simulink model "dstatcom_avg"  (Simulink 7.9)
settings: Solver=ode23tb  SolverMode=SingleTasking  StartTime=0.0  StopTime=12  FixedStep=Ts  MaxStep=1/60  RelTol=1e-4
InitFcn:
  | Ts=40e-6;
  | tic;
StopFcn:
  | toc;
undefined symbols (not defined in the file or in its folder): D11, Delta, DiscIntNeverNeededParam
libraries: powerlib x53, powerlib_extras x39
(part 2 of 2)

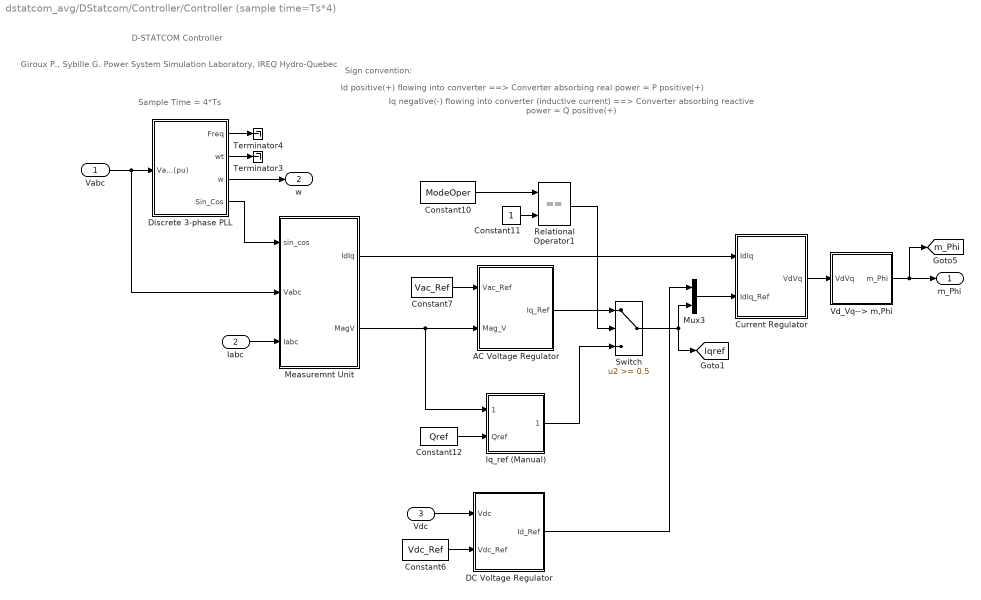
== system dstatcom_avg/DStatcom/Controller/Controller (sample time=Ts*4) ==
  note: D-STATCOM Controller
  note: Giroux P., Sybille G.
      | Power System Simulation Laboratory, IREQ
      | Hydro-Quebec
  note: Iq negative(-) flowing into converter (inductive current) ==> Converter absorbing reactive power = Q positive(+)
  note: Sign convention:
  note: Id positive(+) flowing into converter ==> Converter absorbing real power = P positive(+)
  note: Sample Time = 4*Ts
  Vabc : Inport  PortDimensions=3
  Iabc : Inport  Port=2  PortDimensions=3
  Vdc : Inport  Port=3  PortDimensions=1
  AC Voltage Regulator : Subsystem  mask(DC Voltage regulator){Kp=Kp_Vac, Ki=Ki_Vac, Ts=4*Ts}
      mask prompts: Kp "Proportional gain (Kp):"; Ki "Integral gain(Ki)"; Ts "Sample time:"
  Constant10 : Constant  Value=ModeOper
  Constant11 : Constant
  Constant12 : Constant  Value=Qref
  Constant6 : Constant  Value=Vdc_Ref
  Constant7 : Constant  Value=Vac_Ref
  Current Regulator : Subsystem  mask(Current Regulators){Kp=Kp_I, Ki=Ki_I, Kd=Kd_I, TcD=0.2e-3, Par_Limits=[1 -1], Init=0, Ts=4*Ts}
      mask prompts: Kp "Proportional gain (Kp):"; Ki "Integral gain (Ki):"; Kd "Derivative gain (Kd):"; TcD "Time constant for derivative (s):"; Par_Limits "Output limits: [ Upper   Lower ]"; Init "Output initial value:"; Ts "Sample time:"
      mask help:
      | Sign convention:
      | Id positive(+) flowing into converter ==> Converter absorbing real power = P positive(+)
      | Iq negative(-) flowing into converter (inductive current) ==> Converter absorbing reactive power = Q positive(+)
  DC Voltage Regulator : Subsystem  mask(DC Voltage regulator){Kp=Kp_Vdc, Ki=Ki_Vdc, Ts=4*Ts}
      mask prompts: Kp "Proportional gain (Kp):"; Ki "Integral gain(Ki)"; Ts "Sample time:"
  Discrete 3-phase PLL : Subsystem  mask(Discrete 3-phase PLL){Par_Init=[3.7 60], ParK=[60 1400], Ts=4*Ts}
      mask prompts: Par_Init "Initial inputs:[ Phase(degrees)   Frequency(Hz) ]"; ParK "Regulator gains [ Kp  Ki ]"; Ts "Sample time:"
      mask help:
      | This Phase Locked Loop (PLL) system can be used  to synchronize on a set of variable frequency, three-phase sinusoidal signals.
      |
      | Input 1: Vector containing the normalized
      |              three-phase signals [Va Vb Vc]
      | Output 1:  Measured frequency (Hz) = w/(2pi)
      | Output 2:  Ramp w.t   varying between  0 and 2*pi,
      | synchronized on zero crossings of the fundamental (positive-sequence) of phase A.
      | Output 3: Vector [sin(wt) cos(wt)]
      mask init:
      | Kp=ParK(1);
      | Ki=ParK(2);
      | Phase_Init=Par_Init(1);
      | Finit=Par_Init(2);
  Iq_ref (Manual) : Subsystem
  Measuremnt Unit : Subsystem
  Mux3 : Mux  Inputs=2
  Relational Operator1 : RelationalOperator  Operator===  InputSameDT=on
  Switch : Switch  Threshold=0.5  SaturateOnIntegerOverflow=on  InputSameDT=on
  Terminator3 : Terminator
  Terminator4 : Terminator
  Vd_Vq--> m,Phi : Subsystem
  m_Phi : Outport
  w : Outport  Port=2
  tag scope: Iqref=global, m_Phi=global
  wires:
  Vd_Vq--> m,Phi/1(m_Phi) -> [m_Phi], m_Phi/1
  Current Regulator/1(VdVq) -> Vd_Vq--> m,Phi/1(VdVq)
  Relational Operator1/1 -> Switch/2
  Iq_ref (Manual)/1(Iqref*) -> Switch/3
  DC Voltage Regulator/1(Id_Ref) -> Mux3/1
  Switch/1 -> [Iqref], Mux3/2
  Mux3/1 -> Current Regulator/2(IdIq_Ref)
  AC Voltage Regulator/1(Iq_Ref) -> Switch/1
  Measuremnt Unit/1(IdIq) -> Current Regulator/1(IdIq)
  Constant7/1 -> AC Voltage Regulator/1(Vac_Ref)
  Measuremnt Unit/2(MagV) -> Iq_ref (Manual)/1(MagV), AC Voltage Regulator/2(Mag_V)
  Iabc/1 -> Measuremnt Unit/3(Iabc)
  Discrete 3-phase PLL/4(Sin_Cos) -> Measuremnt Unit/1(sin_cos)
  Discrete 3-phase PLL/3(w) -> w/1
  Discrete 3-phase PLL/1(Freq) -> Terminator4/1
  Discrete 3-phase PLL/2(wt) -> Terminator3/1
  Constant12/1 -> Iq_ref (Manual)/2(Qref)
  Constant10/1 -> Relational Operator1/1
  Constant11/1 -> Relational Operator1/2
  Vdc/1 -> DC Voltage Regulator/1(Vdc)
  Constant6/1 -> DC Voltage Regulator/2(Vdc_Ref)
  Vabc/1 -> Measuremnt Unit/2(Vabc), Discrete 3-phase PLL/1(Vabc (pu))

== system dstatcom_avg/DStatcom/Controller/m_Phi->Vabc(t) ==
  m_Phi : Inport
  theta : Inport  Port=2
  Constant1 : Constant  Value=[0 -2*pi/3 2*pi/3]
  Demux : Demux  Outputs=2
  Product2 : Product  SaturateOnIntegerOverflow=on  InputSameDT=on  OutDataTypeStr=Inherit: Same as first input
  Sum4 : Sum  Inputs=+++  SaturateOnIntegerOverflow=on  InputSameDT=on  OutDataTypeStr=Inherit: Same as first input
  Trigonometric Function1 : Trigonometry
  deg. ->rad : Gain  Gain=pi/180  SaturateOnIntegerOverflow=on  OutDataTypeStr=Inherit: Same as input  ParamDataTypeStr=Inherit: Same as input
  Vabc (t) : Outport
  wires:
  Demux/2 -> deg. ->rad/1
  theta/1 -> Sum4/3
  deg. ->rad/1 -> Sum4/1
  m_Phi/1 -> Demux/1
  Product2/1 -> Vabc (t)/1
  Demux/1 -> Product2/1
  Constant1/1 -> Sum4/2
  Sum4/1 -> Trigonometric Function1/1
  Trigonometric Function1/1 -> Product2/2

== system dstatcom_avg/DStatcom/Controller/w->theta ==
  w : Inport
  Constant4 : Constant  Value=2*pi
  Discrete-Time Integrator : DiscreteIntegrator  SampleTime=Ts  ICPrevOutput=DiscIntNeverNeededParam  ICPrevScaledInput=DiscIntNeverNeededParam
  Math Function : Math  Operator=mod  SaturateOnIntegerOverflow=on
  theta : Outport
  wires:
  Math Function/1 -> theta/1
  w/1 -> Discrete-Time Integrator/1
  Constant4/1 -> Math Function/2
  Discrete-Time Integrator/1 -> Math Function/1

== system dstatcom_avg/DStatcom/Controller/Controller (sample time=Ts*4)/AC Voltage Regulator ==
  Vac_Ref : Inport
  Mag_V : Inport  Port=2
  Discrete PI Controller : powerlib_extras/Discrete  Control Blocks/Discrete PI Controller  Kp=Kp  Ki=Ki  Par_Limits=[1 -1]  Init=0  Ts=Ts
  Sum : Sum  Inputs=|+-  SaturateOnIntegerOverflow=on  InputSameDT=on  OutDataTypeStr=Inherit: Same as first input
  Iq_Ref : Outport  InitialOutput=0
  wires:
  Sum/1 -> Discrete PI Controller/1
  Vac_Ref/1 -> Sum/1
  Mag_V/1 -> Sum/2
  Discrete PI Controller/1 -> Iq_Ref/1

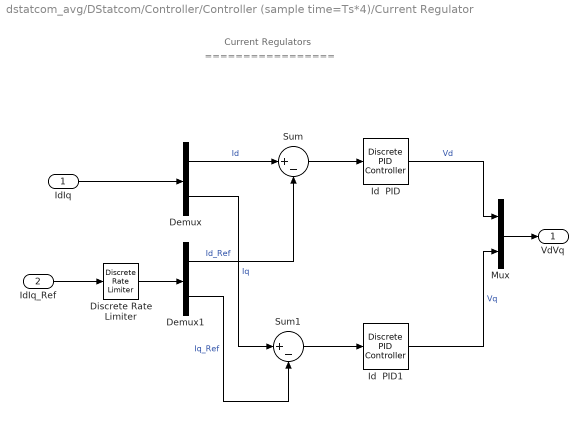
== system dstatcom_avg/DStatcom/Controller/Controller (sample time=Ts*4)/Current Regulator ==
  note: =================
  note: Current Regulators
  IdIq : Inport  PortDimensions=2
  IdIq_Ref : Inport  Port=2  PortDimensions=2
  Demux : Demux  Outputs=2
  Demux1 : Demux  Outputs=2
  Discrete Rate Limiter : powerlib_extras/Discrete  Control Blocks/Discrete Rate Limiter  R=240  F=-240  Vinit=0  Ts=Ts
  Id  PID : powerlib_extras/Discrete  Control Blocks/Discrete PID Controller  Kp=Kp  Ki=Ki  Kd=Kd  TcD=TcD  Par_Limits=Par_Limits  Init=Init  Ts=Ts
  Id  PID1 : powerlib_extras/Discrete  Control Blocks/Discrete PID Controller  Kp=Kp  Ki=Ki  Kd=Kd  TcD=TcD  Par_Limits=Par_Limits  Init=Init  Ts=Ts
  Mux : Mux  Inputs=2
  Sum : Sum  Inputs=|+-  SaturateOnIntegerOverflow=on  InputSameDT=on  OutDataTypeStr=Inherit: Same as first input
  Sum1 : Sum  Inputs=|+-  SaturateOnIntegerOverflow=on  InputSameDT=on  OutDataTypeStr=Inherit: Same as first input
  VdVq : Outport
  wires:
  Discrete Rate Limiter/1 -> Demux1/1
  IdIq_Ref/1 -> Discrete Rate Limiter/1
  Mux/1 -> VdVq/1
  Sum/1 -> Id  PID/1
  Demux1/2 -> Sum1/2  "Iq_Ref"
  Sum1/1 -> Id  PID1/1
  Demux/2 -> Sum1/1  "Iq"
  Demux1/1 -> Sum/2  "Id_Ref"
  Demux/1 -> Sum/1  "Id"
  Id  PID/1 -> Mux/1  "Vd"
  Id  PID1/1 -> Mux/2  "Vq"
  IdIq/1 -> Demux/1

== system dstatcom_avg/DStatcom/Controller/Controller (sample time=Ts*4)/DC Voltage Regulator ==
  Vdc : Inport
  Vdc_Ref : Inport  Port=2
  -1<Id<+1 : Saturate  UpperLimit=1  LowerLimit=-1
  2250<Vdc<3750 : Saturate  UpperLimit=3750  LowerLimit=2250
  Discrete PI Controller : powerlib_extras/Discrete  Control Blocks/Discrete PI Controller  Kp=Kp  Ki=Ki  Par_Limits=[1 -1]  Init=0  Ts=Ts
  Discrete Rate Limiter1 : powerlib_extras/Discrete  Control Blocks/Discrete Rate Limiter  R=10000  F=-10000  Vinit=3000  Ts=Ts
  Sum : Sum  Inputs=|+-  SaturateOnIntegerOverflow=on  InputSameDT=on  OutDataTypeStr=Inherit: Same as first input
  Id_Ref : Outport  InitialOutput=0
  wires:
  Vdc_Ref/1 -> 2250<Vdc<3750/1
  2250<Vdc<3750/1 -> Discrete Rate Limiter1/1
  Sum/1 -> Discrete PI Controller/1
  Vdc/1 -> Sum/2
  Discrete Rate Limiter1/1 -> Sum/1
  Discrete PI Controller/1 -> -1<Id<+1/1
  -1<Id<+1/1 -> Id_Ref/1

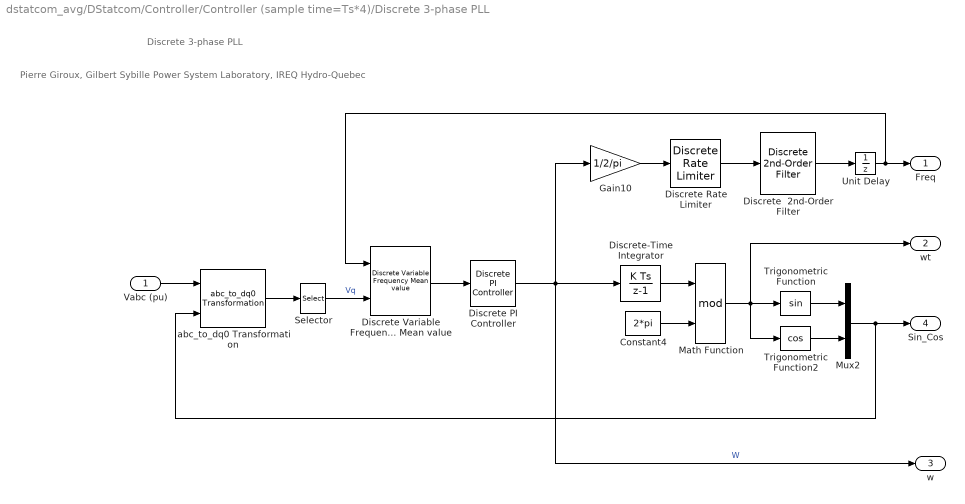
== system dstatcom_avg/DStatcom/Controller/Controller (sample time=Ts*4)/Discrete 3-phase PLL ==
  note: Discrete 3-phase PLL
  note: Pierre Giroux, Gilbert Sybille
      | Power System Laboratory, IREQ
      | Hydro-Quebec
  Vabc (pu) : Inport  PortDimensions=3
  Constant4 : Constant  Value=2*pi
  Discrete PI Controller : powerlib_extras/Discrete  Control Blocks/Discrete PI Controller  Kp=Kp  Ki=Ki  Par_Limits=2*pi*Finit*[1.25 0.75]  Init=2*pi*Finit  Ts=Ts
  Discrete Rate Limiter : powerlib_extras/Discrete  Control Blocks/Discrete Rate Limiter  R=10  F=-10  Vinit=Finit  Ts=Ts
  Discrete Variable Frequency Mean value : powerlib_extras/Discrete Measurements/Discrete Variable Frequency Mean value  Finit=Finit  Fmin=45  Vinit=0  Ts=Ts
  Discrete  2nd-Order Filter : powerlib_extras/Discrete  Control Blocks/Discrete  2nd-Order Filter  FilterType=Lowpass  Fo=25  Zeta=0.707  Ts=Ts  Initialize=on  Vac_Init=[0 0 Finit]  Vdc_Init=Finit  PlotResponse=off  param1=[1 500 0.1]
  Discrete-Time Integrator : DiscreteIntegrator  InitialCondition=Phase_Init*pi/180  SampleTime=Ts  ICPrevOutput=DiscIntNeverNeededParam  ICPrevScaledInput=DiscIntNeverNeededParam
  Gain10 : Gain  Gain=1/2/pi  SaturateOnIntegerOverflow=on  OutDataTypeStr=Inherit: Same as input  ParamDataTypeStr=Inherit: Same as input
  Math Function : Math  Operator=mod  SaturateOnIntegerOverflow=on
  Mux2 : Mux  Inputs=2
  Selector : Selector  InputPortWidth=3  IndexOptions=Index vector (dialog)  Indices=2  OutputSizes=1
  Trigonometric Function : Trigonometry
  Trigonometric Function2 : Trigonometry  Operator=cos
  Unit Delay : UnitDelay  X0=Finit  SampleTime=Ts
  abc_to_dq0 Transformation : powerlib_extras/Measurements/abc_to_dq0 Transformation
  Freq : Outport
  wt : Outport  Port=2
  w : Outport  Port=3
  Sin_Cos : Outport  Port=4
  wires:
  Discrete Variable Frequency Mean value/1 -> Discrete PI Controller/1
  Vabc (pu)/1 -> abc_to_dq0 Transformation/1
  abc_to_dq0 Transformation/1 -> Selector/1
  Constant4/1 -> Math Function/2
  Discrete-Time Integrator/1 -> Math Function/1
  Math Function/1 -> Trigonometric Function/1, Trigonometric Function2/1, wt/1
  Trigonometric Function/1 -> Mux2/1
  Trigonometric Function2/1 -> Mux2/2
  Mux2/1 -> abc_to_dq0 Transformation/2, Sin_Cos/1
  Discrete PI Controller/1 -> w/1, Discrete-Time Integrator/1, Gain10/1  "W"
  Gain10/1 -> Discrete Rate Limiter/1
  Discrete Rate Limiter/1 -> Discrete  2nd-Order Filter/1
  Unit Delay/1 -> Freq/1, Discrete Variable Frequency Mean value/1
  Discrete  2nd-Order Filter/1 -> Unit Delay/1
  Selector/1 -> Discrete Variable Frequency Mean value/2  "Vq"

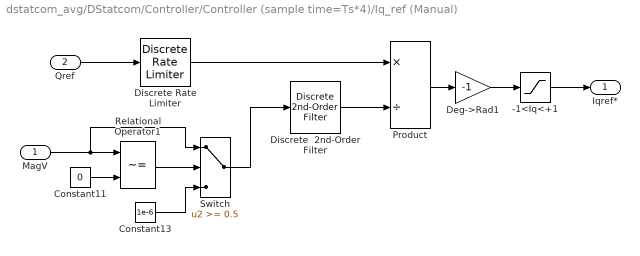
== system dstatcom_avg/DStatcom/Controller/Controller (sample time=Ts*4)/Iq_ref (Manual) ==
  MagV : Inport  PortDimensions=1
  Qref : Inport  Port=2  PortDimensions=1
  -1<Iq<+1 : Saturate  UpperLimit=1  LowerLimit=-1
  Constant11 : Constant  Value=0
  Constant13 : Constant  Value=1e-6
  Deg->Rad1 : Gain  Gain=-1  SaturateOnIntegerOverflow=on  OutDataTypeStr=Inherit: Same as input  ParamDataTypeStr=Inherit: Same as input
  Discrete Rate Limiter : powerlib_extras/Discrete  Control Blocks/Discrete Rate Limiter  R=60*2  F=-60*2  Vinit=0  Ts=4*Ts
  Discrete  2nd-Order Filter : powerlib_extras/Discrete  Control Blocks/Discrete  2nd-Order Filter  FilterType=Lowpass  Fo=20  Zeta=0.707  Ts=4*Ts  Initialize=off  Vac_Init=[0.8 -25 60]  Vdc_Init=-0.4  PlotResponse=off  param1=[1 500 0.1]
  Product : Product  Inputs=*/  SaturateOnIntegerOverflow=on  InputSameDT=on  OutDataTypeStr=Inherit: Same as first input
  Relational Operator1 : RelationalOperator  Operator=~=  InputSameDT=on
  Switch : Switch  Threshold=0.5  SaturateOnIntegerOverflow=on  InputSameDT=on
  Iqref* : Outport
  wires:
  Discrete Rate Limiter/1 -> Product/1
  Qref/1 -> Discrete Rate Limiter/1
  -1<Iq<+1/1 -> Iqref*/1
  Deg->Rad1/1 -> -1<Iq<+1/1
  Product/1 -> Deg->Rad1/1
  Discrete  2nd-Order Filter/1 -> Product/2
  Switch/1 -> Discrete  2nd-Order Filter/1
  Constant13/1 -> Switch/3
  MagV/1 -> Switch/1, Relational Operator1/1
  Relational Operator1/1 -> Switch/2
  Constant11/1 -> Relational Operator1/2

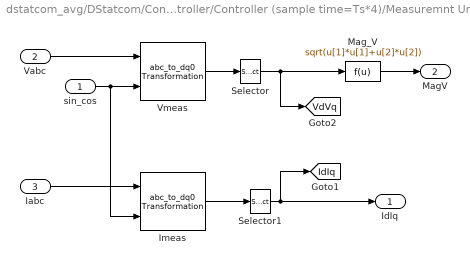
== system dstatcom_avg/DStatcom/Controller/Controller (sample time=Ts*4)/Measuremnt Unit ==
  sin_cos : Inport
  Vabc : Inport  Port=2
  Iabc : Inport  Port=3
  Imeas : powerlib_extras/Measurements/abc_to_dq0 Transformation
  "Mag_V " : Fcn  Expr=sqrt(u[1]*u[1]+u[2]*u[2])
  Selector : Selector  InputPortWidth=3  IndexOptions=Index vector (dialog)  Indices=[1 2]  OutputSizes=1
  Selector1 : Selector  InputPortWidth=3  IndexOptions=Index vector (dialog)  Indices=[1 2]  OutputSizes=1
  Vmeas : powerlib_extras/Measurements/abc_to_dq0 Transformation
  IdIq : Outport
  MagV : Outport  Port=2
  tag scope: IdIq=global, VdVq=global
  wires:
  "Mag_V "/1 -> MagV/1
  Selector1/1 -> [IdIq], IdIq/1
  Selector/1 -> "Mag_V "/1, [VdVq]
  Imeas/1 -> Selector1/1
  Iabc/1 -> Imeas/1
  sin_cos/1 -> Imeas/2, Vmeas/2
  Vmeas/1 -> Selector/1
  Vabc/1 -> Vmeas/1

== system dstatcom_avg/DStatcom/Controller/Controller (sample time=Ts*4)/Vd_Vq--> m,Phi ==
  VdVq : Inport
  Fcn3 : Fcn  Expr=sqrt(u[1]*u[1]+u[2]*u[2])
  Fcn4 : Fcn  Expr=atan2(u[2]+1e-6,u[1])*180/pi
  Mux2 : Mux  Inputs=2
  m_Phi : Outport
  wires:
  Fcn4/1 -> Mux2/2
  Mux2/1 -> m_Phi/1
  Fcn3/1 -> Mux2/1
  VdVq/1 -> Fcn4/1, Fcn3/1
